simulink model "CMU_BORG_AplysiaModularNeuromechanics"  (R2024a)
settings: Solver=ode23  StartTime=0.0  StopTime=tend  FixedStep=0.001  MaxStep=0.1  RelTol=0.00001  AbsTol=0.0001
values from neighbouring files (symbols this model uses):
  B20_0 = 0    [ParameterRecalculation.m]    (also in ReferenceGeometry_and_Initialization.m)
  B31B32_0 = 0    [GetSteadyState.m]    (also in ParameterRecalculation.m = 1; ReferenceGeometry_and_Initialization.m = 1; VaryingSeaweedStrength.m = 1)
  B38_0 = 0    [ParameterRecalculation.m]    (also in ReferenceGeometry_and_Initialization.m)
  B40B30_0 = 0    [ParameterRecalculation.m]    (also in ReferenceGeometry_and_Initialization.m)
  B40B30_offTime_0 = 0    [ParameterRecalculation.m]    (also in ReferenceGeometry_and_Initialization.m)
  B43B45_0 = 0    [ParameterRecalculation.m]    (also in ReferenceGeometry_and_Initialization.m)
  B4B5_0 = 0    [ParameterRecalculation.m]    (also in ReferenceGeometry_and_Initialization.m)
  B64_0 = 1    [GetSteadyState.m]    (also in ParameterRecalculation.m = 0; ReferenceGeometry_and_Initialization.m = 0; VaryingSeaweedStrength.m = 0)
  B6B9B3_0 = 1    [GetSteadyState.m]    (also in ParameterRecalculation.m = 0; ReferenceGeometry_and_Initialization.m = 0; VaryingSeaweedStrength.m = 0)
  B7_0 = 0    [ParameterRecalculation.m]    (also in ReferenceGeometry_and_Initialization.m)
  B8_0 = 0    [ParameterRecalculation.m]    (also in ReferenceGeometry_and_Initialization.m)
  C1_0 = 0    [ParameterRecalculation.m]    (also in ReferenceGeometry_and_Initialization.m)
  C2_0 = 0    [ParameterRecalculation.m]    (also in ReferenceGeometry_and_Initialization.m)
  C6_0 = 0    [ParameterRecalculation.m]    (also in ReferenceGeometry_and_Initialization.m)
  C_theta = C_xg/(2*pi)    [ParameterRecalculation.m]    (also in ReferenceGeometry_and_Initialization.m = 0.000813600069086)
  C_xd = C_xg    [ParameterRecalculation.m]    (also in ReferenceGeometry_and_Initialization.m = 0.005112)
  C_xg = (1/inv_C(kk))*time_scaler*force_scaler    [DampingParameterConvergence.m]    (also in ReferenceGeometry_and_Initialization.m = 0.005112)
  C_xv = C_xd    [ParameterRecalculation.m]    (also in ReferenceGeometry_and_Initialization.m = 0.005112)
  C_yg = C_xg    [ParameterRecalculation.m]    (also in ReferenceGeometry_and_Initialization.m = 0.005112)
  CBI2_0 = 0    [ParameterRecalculation.m]    (also in ReferenceGeometry_and_Initialization.m)
  CBI3_0 = 0    [GetSteadyState.m]    (also in ParameterRecalculation.m = 1; ReferenceGeometry_and_Initialization.m = 1; VaryingSeaweedStrength.m = 1)
  CBI3_refractory_0 = 0    [ParameterRecalculation.m]    (also in ReferenceGeometry_and_Initialization.m)
  CBI3_stimOFF_0 = 0    [ParameterRecalculation.m]    (also in ReferenceGeometry_and_Initialization.m)
  CBI3_stimON_0 = 0    [ParameterRecalculation.m]    (also in ReferenceGeometry_and_Initialization.m)
  CBI4_0 = 0    [ParameterRecalculation.m]    (also in ReferenceGeometry_and_Initialization.m)
  E1_params = [AE10,TE10,tau_E1,L0_E1,Lmax_E1]    [ParameterRecalculation.m]    (also in ReferenceGeometry_and_Initialization.m)
  E2_params = [AE20,TE20,tau_E2,L0_E2,Lmax_E2]    [ParameterRecalculation.m]    (also in ReferenceGeometry_and_Initialization.m)
  E6_params = [AE60,TE60,tau_E6,L0_E6,Lmax_E6]    [ParameterRecalculation.m]    (also in ReferenceGeometry_and_Initialization.m)
  FE1_max = force_scaler*0.2    [ParameterRecalculation.m]    (also in ReferenceGeometry_and_Initialization.m = 0.048)
  FE2_max = FE1_max    [ParameterRecalculation.m]    (also in ReferenceGeometry_and_Initialization.m = 0.048)
  FE6_max = FE1_max    [ParameterRecalculation.m]    (also in ReferenceGeometry_and_Initialization.m = 0.048)
  FHinge_max = force_scaler*0.292    [ParameterRecalculation.m]    (also in ReferenceGeometry_and_Initialization.m = 0.07008)
  FI1d_max = force_scaler*3.2    [ParameterRecalculation.m]    (also in ReferenceGeometry_and_Initialization.m = 0.768)
  FI1v_max = FI1d_max    [ParameterRecalculation.m]    (also in ReferenceGeometry_and_Initialization.m = 0.768)
  FI2_max = force_scaler*1    [ParameterRecalculation.m]    (also in ReferenceGeometry_and_Initialization.m = 0.24)
  FI3_ant_max = force_scaler*0.1    [ParameterRecalculation.m]    (also in ReferenceGeometry_and_Initialization.m = 0.024)
  FI3_max = force_scaler*3    [ParameterRecalculation.m]    (also in ReferenceGeometry_and_Initialization.m = 0.72)
  FI4_max = force_scaler*0.9    [ParameterRecalculation.m]    (also in ReferenceGeometry_and_Initialization.m = 0.216)
  fixation_type = 0    [GetSteadyState.m]    (also in ModelController.m; VaryingSeaweedStrength.m)
  grasperR = 1    [ReferenceGeometry_and_Initialization.m]
  H_lumen = mean([L_jaw,L_LG]) / R_ref    [ReferenceGeometry_and_Initialization.m]
  Hinge_params = [A_hinge0,T_hinge0,tau_hinge,L0_hinge,Lmax_hinge]    [ParameterRecalculation.m]    (also in ReferenceGeometry_and_Initialization.m)
  I1d_params = [AI1d0,TI1d0,tau_I1d,L0_I1d,Lmax_I1d]    [ParameterRecalculation.m]    (also in ReferenceGeometry_and_Initialization.m)
  I1v_params = [AI1v0,TI1v0,tau_I1v,L0_I1v,Lmax_I1v]    [ParameterRecalculation.m]    (also in ReferenceGeometry_and_Initialization.m)
  I2_params = [AI20,TI20,tau_I2_ingestive,tau_I2_egestive,L0_I2,Lmax_I2]    [ParameterRecalculation.m]    (also in ReferenceGeometry_and_Initialization.m)
  I3_params = [AI30,TI30,tau_I3]    [ParameterRecalculation.m]    (also in ReferenceGeometry_and_Initialization.m)
  I3ant_params = [AI3_ant0,TI3_ant0,tau_I3ant]    [ParameterRecalculation.m]    (also in ReferenceGeometry_and_Initialization.m)
  I4_params = [AI40,TI40,tau_I4]    [ParameterRecalculation.m]    (also in ReferenceGeometry_and_Initialization.m)
  K_const = force_scaler*0.5    [ParameterRecalculation.m]    (also in ReferenceGeometry_and_Initialization.m = 0.12)
  K_Eso = force_scaler*0.01    [ParameterRecalculation.m]    (also in ReferenceGeometry_and_Initialization.m = 0.0024)
  K_H = force_scaler*2    [ParameterRecalculation.m]    (also in ReferenceGeometry_and_Initialization.m = 0.48)
  L0_eso = abs(xd0)    [ReferenceGeometry_and_Initialization.m]
  L0_H = 0    [ReferenceGeometry_and_Initialization.m]
  L0_I1d = L1d0    [ParameterRecalculation.m]    (also in ReferenceGeometry_and_Initialization.m)
  L0_I1v = L1v0    [ParameterRecalculation.m]    (also in ReferenceGeometry_and_Initialization.m)
  L_head = 0.82*tracing_scale_factor    [ReferenceGeometry_and_Initialization.m]
  MCC_0 = 1    [DampingParameterConvergence.m]    (also in ModelController.m; ParameterRecalculation.m = 0; ReferenceGeometry_and_Initialization.m = 0)
  params = param_vec    [ParameterRecalculation.m]    (also in ReferenceGeometry_and_Initialization.m)
  seaweed_strength = 1e6    (= 1000000)    [ModelController.m]    (also in VaryingSeaweedStrength.m = seaweed_strength_vec(ind))
  sens_chemical_lips = 0    [GetSteadyState.m]    (also in ModelController.m = 1; VaryingSeaweedStrength.m = 1)
  sens_mechanical_grasper = 1    [GetSteadyState.m]    (also in ModelController.m = 0; VaryingSeaweedStrength.m)
  sens_mechanical_lips = 1    [GetSteadyState.m]    (also in ModelController.m; VaryingSeaweedStrength.m)
  t_switch_chem_lips = 1e6    (= 1000000)    [GetSteadyState.m]    (also in ModelController.m = 54; VaryingSeaweedStrength.m)
  t_switch_fixation = 1e6    (= 1000000)    [GetSteadyState.m]    (also in ModelController.m = 30; VaryingSeaweedStrength.m = 4)
  t_switch_mech_grasp = 1e6    (= 1000000)    [GetSteadyState.m]    (also in ModelController.m = 10; VaryingSeaweedStrength.m)
  t_switch_mech_lips = 1e6    (= 1000000)    [GetSteadyState.m]    (also in ModelController.m; VaryingSeaweedStrength.m)
  theta_fg = buccal_mass_data(7)    [PlotModel.m]    (also in ReferenceGeometry_and_Initialization.m = -(head_outline{4,"Angle"} - head_outline{3,"Angle"})*(pi/180)
  theta_g0 = (180-(head_outline{3,"Angle"} + rot_global +5))*(pi/180)    [ReferenceGeometry_and_Initialization.m]
  theta_H = buccal_mass_data(6)    [PlotModel.m]    (also in ReferenceGeometry_and_Initialization.m = pi + theta_H_tilde - theta_g0)
  time_scaler = 1    [DampingParameterConvergence.m]    (also in ReferenceGeometry_and_Initialization.m = 1.065)
  ukg = 0.95*usg    (= 0.95)    [ParameterRecalculation.m]    (also in ReferenceGeometry_and_Initialization.m)
  ukh = 0.75*ush    (= 0.75)    [ParameterRecalculation.m]    (also in ReferenceGeometry_and_Initialization.m)
  usg = 1    [ParameterRecalculation.m]    (also in ReferenceGeometry_and_Initialization.m)
  ush = 1    [ParameterRecalculation.m]    (also in ReferenceGeometry_and_Initialization.m)
  xd0 = L_head - L1d0    [ReferenceGeometry_and_Initialization.m]
  xg0 = L_head + L_CG * cosd(a_CG) + 0.3    [ReferenceGeometry_and_Initialization.m]
  xh0 = 0    [ReferenceGeometry_and_Initialization.m]
  xv0 = L_head - L1v0    [ReferenceGeometry_and_Initialization.m]
  yg0 = L_CG * sind(a_CG) + 0.4    [ReferenceGeometry_and_Initialization.m]
(part 4 of 4)

== matlab function CMU_BORG_AplysiaModularNeuromechanics/Neural Model Module Webster-Wood et al. 1/MATLAB Function ==
  data: CBI3_stimOFF output; CBI3_refractory output; B40B30 output; Time input; time_scaler input; MCC output; stim_CBI2_old input; stim_B4B5_old input; sens_mechanical_lips_old input; sens_chemical_lips_old input; sens_mechanical_grasper_old input; CBI3_stimOFF_old input; CBI3_refractory_old input; B40B30_old input; CBI2 output; MCC_old input; CBI2_old input; CBI3_stimON_old input; CBI4_old input; B64_old input; B4B5_old input; B20_old input; B40B30_offTime input; CBI3_old input; B31B32_old input; P_I4_old input; x_gh input; CBI3_stimON output; CBI4 output; B64 output; B4B5 output; B20 output; B40B30_offTime output; B8 output; B38 output; B6B9B3 output; CBI3 output; B31B32 output; B7 output; params input
function [CBI3_stimOFF, CBI3_refractory, B40B30, MCC, CBI2, CBI3_stimON, CBI4, B64, B4B5, B20, B40B30_offTime, B8, B38, B6B9B3, CBI3, B31B32, B7]...
    = neuromechanics(Time,time_scaler, stim_CBI2_old, stim_B4B5_old, sens_mechanical_lips_old, sens_chemical_lips_old, sens_mechanical_grasper_old,...
    CBI3_stimOFF_old, CBI3_refractory_old, B40B30_old, MCC_old, CBI2_old, CBI3_stimON_old, ...
    CBI4_old, B64_old, B4B5_old, B20_old, B40B30_offTime, CBI3_old, B31B32_old, ...
    P_I4_old, x_gh, params)

    % All time related values were changed from step-number-dependent to
    % actual simulation time dependent for compatibility with variable
    % time-step solvers. --MB

    %% Parameter definition based on the params vector
    thresh_B31_bite_off =            params(1) ;  % retraction level at which to turn I2 back on
    thresh_B64_bite_protract =       params(2) ; % protraction level at which to turn I3 on (once I2 turns off)
    thresh_B31_bite_on =             params(3) ;  % protraction level at which to turn I2 off
    thresh_B7_bite_protract =        params(4) ;  % protraction level at which to turn the hinge on
    thresh_B7_bite_pressure =        params(5) ;   % pressure level at which B7 turns on
    thresh_B6B9B3_bite_pressure =    params(6) ;  % pressure threshold needed before I3 turns on 
    thresh_B31_pressure_bite =       params(7) ;
    
    thresh_B64_swallow_protract =    params(8) ;  % protraction level above which to turn on I3
    thresh_B31_swallow_off =         params(9) ; % retraction level at which to turn I2 back on 
    thresh_B31_swallow_on =          params(10) ;
    thresh_B6B9B3_swallow_pressure = params(11) ;
    thresh_B38_retract =             params(12) ;
    thresh_B31_pressure_swallow =    params(13) ;
    
    % rejection params
    thresh_B64_reject_protract =     params(14) ;
    thresh_B4B5_protract =           params(15) ;
    thresh_B31_reject_off =          params(16) ;
    thresh_B31_reject_on =           params(17) ;
    thresh_B7_reject_protract =      params(18) ;
    thresh_B7_reject_pressure =      params(19) ;   % pressure level at which B7 turns on
    thresh_B6B9B3_reject_pressure =  params(20) ;
    thresh_B31_pressure_reject =     params(21) ;
    refractory_CBI3 = params(22) ;
    
    postActivityExcitation_B40B30 = params(23);

    %switches
    use_hypothesized_connections = 1; %1 = yes, 0 = no

%% Update Metacerebral cell: 
                % assume here feeding arousal continues
                % indefinitely, once started. 
                %{
                MCC is active IF
                    General Food arousal is on
                %}

                MCC = MCC_old;    
    %% Update CBI-2
    
    %CBI2 - updated 6/7/2020
    %with hypothesized connections from B4/B5
    %%%%% MJB 5/27/2025 The second row of the condition (for rejection) was
    %%%%% missing the negation in front of the chemical lip stimulation.
    if (use_hypothesized_connections ==1)
         CBI2 = (stim_CBI2_old==0)*... if electrode above CBI-2 is off, do this:
             MCC_old*(~B64_old)*( (sens_mechanical_lips_old && sens_chemical_lips_old &&(~sens_mechanical_grasper_old)) || ...
                                  (sens_mechanical_grasper_old &&(~sens_chemical_lips_old)) || ...
                                  (B4B5_old>=2) )+...
             (stim_CBI2_old==1);
    else
    %without hypothesized connections from B4/B5
        CBI2 = (stim_CBI2_old==0)*... if electrode above CBI-2 is off, do this:
            MCC_old*(~B64_old)*((sens_mechanical_lips_old && sens_chemical_lips_old &&(~sens_mechanical_grasper_old))||(sens_mechanical_grasper_old&&(~sens_chemical_lips_old)))+...
            (stim_CBI2_old==1);
    end

    
    %% Update CBI-3
    
            % requires stimuli_mech_last AND stimuli_chem_last
        %{
        CBI3 is active IF
            MCC is on
            AND
            Mechanical Simulation at Lips
            AND
            Chemical Stimulation at Lips
            AND
            B4/B5 is NOT firing strongly
            AND
            CBI3 is NOT in a refractory period
        %}

        %CBI3 can experieince a refractory period following strong inhibition from B4/B5
        %check if a refractory period is occuring

    %modified to only turn on refreactory after the strong stimulation
    
        CBI3_refractory = CBI3_refractory_old;
        CBI3_stimOFF = CBI3_stimOFF_old;
        CBI3_stimON = CBI3_stimON_old;
            
        if((B4B5_old>=2) && (CBI3_stimON_old==0))
           CBI3_stimON = Time;   
           %CBI3_refractory = 1;
        end
        

        if ((CBI3_stimON_old ~=0) && (B4B5_old<2))
           CBI3_refractory = 1;
           CBI3_stimOFF = Time;  
           CBI3_stimON = 0;    
        end
        

        if(CBI3_refractory && Time<(CBI3_stimOFF + refractory_CBI3))
           CBI3_refractory = 1; 
        else
            CBI3_stimOFF = 0;
            CBI3_refractory = 0; 
        end


        %CBI3 - updated 6/7/2020    
        %with hypothesized connections from B4/B5    
        if (use_hypothesized_connections ==1)
            CBI3 = MCC_old*(sens_mechanical_lips_old*sens_chemical_lips_old)*((B4B5_old<2))*(~CBI3_refractory);   
        else
        %without hypothesized connections from B4/B5  
            CBI3 = MCC_old*(sens_mechanical_lips_old*sens_chemical_lips_old); 
        end
    %% Update CBI4 - added 2/27/2020
    %{
    CBI4 is active IF  mediates swallowing and rejection
        MCC is on
        AND
            (Mechanical Stimulation at Lips
            OR
            Chemical Stimulation at Lips)
        AND
        Mechanical Stimulation in grasper
    %}
    CBI4 = MCC_old*(sens_mechanical_lips_old || sens_chemical_lips_old)*sens_mechanical_grasper_old;
    
    %% Update B64
    % list of inputs
    % Protraction threshold excites
    % grasper pressure excites - still figuring out how to implement
    % retraction threshold inhibits
    % B31/32 inhibits

    %If there is mechanical and chemical stimuli at the lips and there is
    %seaweed in the grasper -> swallow

    %If there is mechanical and chemical stimuli at the lips and there is
    %NOT seaweed in the grasper -> bite

    %If there is not chemical stimuli at the lips but there is mechanical
    %stimuli ->reject

    %{
    B64 is active IF
        MCC is on
        AND
        IF CBI3 is active (ingestion)
            IF mechanical stimulation is in grasper (swallowing)
                Relative Grasper Position is Greater than B64 Swallowing Protraction threshold
            IF mechanical stimulation is NOT in grasper (biting)
                Relative Grasper Position is Greater than B64 Biting Protraction threshold
        IF CBI3 is NOT active (rejection)
            Relative Grasper Position is Greater than B64 Rejection Protraction threshold
        AND
        B31/B32 is NOT active
        AND
        IF CBI3 is active (ingestion)
            IF mechanical stimulation is in grasper (swallowing)
                NOT (Relative Grasper Position is less than B64 Swallow Retraction threshold)
            IF mechanical stimulation is NOT in grasper (biting)
                NOT(Relative Grasper Position is less than B64 Biting Retraction threshold)
        IF CBI3 is NOT active (rejection)
            NOT(Relative Grasper Position is less than B64 Rejection Retraction threshold)
    %}

    B64_proprioception = (CBI3_old*(... % checks protraction threshold - original 0.5
                                    (  sens_mechanical_grasper_old *(x_gh>thresh_B64_swallow_protract))||...
                                    ((~sens_mechanical_grasper_old)*(x_gh>thresh_B64_bite_protract))))...
                                ||...
                                    ((~CBI3_old)                   *(x_gh>thresh_B64_reject_protract));

    %B64
    B64 = (MCC_old*(~B31B32_old)*B64_proprioception); % update B64
%% Update B4/B5: 
    %{
    B4/B5 is active IF
        MCC is ON
        AND
        IF stimulating electrode is off
            Strongly firing IF CBI3 is NOT active (rejection)
                AND
                B64 is active (retraction)
                AND
                Relative grasper position is greater than B4/B5 threshold (early retraction)
            weakly firing IF CBI3 is active (ingestion)
                AND
                B64 is active (retraction)
                AND
                mechanical stimulation is in grasper (swallowing)
        If stimulating electrode is on
            Activity is set to 2 to designate strong firing
    %}

    %B4B5
    B4B5 = MCC_old*...
                ((~stim_B4B5_old)*... % when B4/B5 electrode is off
                    (2*(~CBI3_old)*...% if egestion
                        B64_old*(x_gh>thresh_B4B5_protract)) +... 
                    ((CBI3_old)*(sens_mechanical_grasper_old)*B64_old))... % if swallowing
        +2*stim_B4B5_old; % when B4/B5 electrode is on (and +1) then turn B4/B5 on to "emergency" mode
    
 %% Update B20 - updated 2/27/2020
    % Not active if CB1-3 is on (strongly inhibited)
    %excited by CBI2 but excitation is weaker than inhibition from CBI3
    %{
    (CBI2 is active
        OR	
        CBI4 is active
        OR
        B63 (B31/32) is active)
            AND
            CBI3 is NOT active
            AND
            B64 is NOT active
    %}
    B20 = MCC_old*((CBI2_old || CBI4_old) || B31B32_old)*(~CBI3_old)*(~B64_old);

%% Update B40/B30
    %{
    B40/B30 is active IF
        MCC is ON
        AND
        (CBI2 is active
        OR 
        CBI4 is active
        OR 
        B63 (B31/32) is active)
        AND 
        B64 is not active
    %}

    % B30/B40 have a fast inhibitory and slow excitatory connection with
    % B8a/b. To accomodate this, we track when B30/B40 goes from a active
    % state to a quiescent state 

    B40B30 = MCC_old*((CBI2_old || CBI4_old) || B31B32_old)*(~B64_old);

    %check if B30/B40 has gone from active to quiescent
    if((B40B30_old == 1) && (B40B30==0))
       B40B30_offTime = Time;
    end
%% Update B31/B32: -updated 2/27/2020
                % activated if grasper retracted enough, inhibited if
                % pressure exceeds a threshold or grasper is protracted far enough
                %{
                B31/B32 is active IF
                    MCC is ON
                    AND
                    IF CBI3 is active (ingestion)
                        B64 is NOT active (protraction)
                        AND
                            Graper pressure is less than half of its maximum (open)
                            OR
                            CBI2 is active (biting)
                        AND
                        IF B31/B32 is NOT firing (switching to protraction)
                            The relative grasper position is less than the retraction threshold
                        IF B31/B32 is firing (protraction)
                            The relative grasper position is less than the protraction threshold
                    IF CBI3 is NOT active (rejection)
                        B64 is NOT active (protraction)
                        AND
                        Grasper Pressure is greater than a quarter of the maximum (closing or closed)
                        AND
                            CBI2 is active
                            OR
                            CBI4 is active
                        AND
                        IF B31/B32 is NOT firing (switching to protraction)
                            The relative grasper position is less than the retraction threshold
                        IF B31/B32 is firing (protraction)
                            The relative grasper position is less than the protraction threshold
                %}

                %B31/B32s thresholds may vary for different behaviors. These are set
                %here
                if (sens_mechanical_grasper_old && CBI3_old) %swallowing
                    on_thresh = thresh_B31_swallow_on;
                    off_thresh = thresh_B31_swallow_off;
                    press_thresh = thresh_B31_pressure_swallow;
                elseif (sens_mechanical_grasper_old && (~CBI3_old)) %rejection
                    on_thresh = thresh_B31_reject_on;
                    off_thresh = thresh_B31_reject_off;
                    press_thresh = thresh_B31_pressure_reject;
                else %biting
                    on_thresh = thresh_B31_bite_on;
                    off_thresh = thresh_B31_bite_off;
                    press_thresh = thresh_B31_pressure_bite;
                end

                B31B32 = MCC_old*(...
                    CBI3_old*... %if ingestion
                        ((~B64_old)*((P_I4_old<(press_thresh))||CBI2_old)*... 
                            ((~B31B32_old)*(x_gh<off_thresh)+...
                               B31B32_old *(x_gh<on_thresh)))+...
                  (~CBI3_old)*... %if egestion
                        ((~B64_old)*(P_I4_old>(press_thresh))*(CBI2_old||CBI4_old)*...
                            ((~B31B32_old)*(x_gh<off_thresh)+...
                               B31B32_old *(x_gh<on_thresh))));

%% Update B6/B9/B3: 
    % activate once pressure is high enough in ingestion, or low enough in
    % rejection
    %{
    NEW VERSION:
    B6/B9/B3 is active IF
        MCC is active
        AND
        B4/B5 is NOT firing strongly
        AND
        IF CBI3 is active (ingestion)
            B64 is active (retraction)
            AND
            Grasper pressure is greater than B6/B3/B9 pressure threshold (closed)
        IF CBI3 is not active (rejection)
            B64 is active (retraction)
            AND
            Grasper pressure is less than B6/B3/B9 pressure threshold (open)
    %}

    %B6/B9/B3
    B6B9B3 = MCC_old*B64_old*(~(B4B5_old>=2))*(...
                    (CBI3_old && ~sens_mechanical_grasper_old)*... biting
                        (P_I4_old>thresh_B6B9B3_bite_pressure)...
                    +...
                    (CBI3_old && sens_mechanical_grasper_old)*... swallowing
                        (P_I4_old>thresh_B6B9B3_swallow_pressure)...
                    +...
                    (~CBI3_old)*... rejection
                        (~(P_I4_old>thresh_B6B9B3_reject_pressure)));

%% Update B8a/b
    % active if excitation from B6/B9/B3 plus protracted
    % sensory feedback exceeds threshold of 1.9, and not inhibited by
    % either B31/B32 or by sensory feedback from being retracted. If B4/B5 is
    % highly excited (activation level is 2 instead of just 1) then shut
    % down B8a/b.
    %{
    B8a/b is active IF
        MCC is on
        AND
            B64 is active
            OR
            B40/B30 is NOT active
            OR
            B20 is active
        AND
        B4/B5 is not active
        AND
            B20 is active
            OR
            B31/B32 is NOT active
    %}

    %B8a/b recieves slow exitatory input from B30/B40 functionally this
    %causes strong firing immediatly following B30/B40 cessation in biting
    %and swallowing
    if(B40B30_old==0 && Time<(B40B30_offTime+postActivityExcitation_B40B30)) %%%%%%%%Changed 'TimeStep' to 0.01 - ASL
        B40B30_excite = 1; 
    else
        B40B30_excite = 0; 
    end

    %B8a/b - updated 5/25/2020   
    B8 = MCC_old*(~(B4B5_old>=2))*(...%B4/5 inhibits when strongly active
                CBI3_old*(... % if ingestion
                    B20_old || (B40B30_excite)*(~B31B32_old))+...
                (~CBI3_old)*(... % if rejection
                    B20_old));                     

%% Update B7 - ONLY ACTIVE DURING EGESTION and BITING
    % turn on as you get to peak protraction
    %in biting this has a threshold that it stops applying effective force -
    %biomechanics
    %{
    B7 is active IF
        ((CBI3 is NOT active (rejection)
        OR
        There is mechanical stimulation in mouth
        AND
            (The relative position of the grasper is greater than the rejection protraction threshold
            OR
            Grasper pressure is very high) (closed))
        OR
        (CBI3 is active
        AND
        There is NOT mechanical stimulation in mouth (biting)
        AND
            (The relative position of the grasper is greater than the bite protraction threshold
            OR
            Grasper pressure is very high) (closed))
    %}
    B7 = MCC_old*( ...
                      (((~CBI3_old) ||  (sens_mechanical_grasper_old))*((x_gh>=thresh_B7_reject_protract)||(P_I4_old>(thresh_B7_reject_pressure)))) + ...
                      (  (CBI3_old  && (~sens_mechanical_grasper_old))*((x_gh>=thresh_B7_bite_protract)  ||(P_I4_old>(thresh_B7_bite_pressure)))) ...
                      );                    

%% Update B38: 
    % If already active, remain active until protracted past
    % 0.5.  If inactive, become active if retracted to 0.1 or further. 
    %{
    B38 is active IF
        MCC is ON
        AND
        mechanical stimulation in the grasper (swallowing or rejection)
        AND
        IF CBI3 is active (ingestion)
            Relative grasper position is less than B38 ingestion threshold
        IF CBI3 is not active (rejection)
            Turn off B38
    %}

    %B38

    B38 = MCC_old*(sens_mechanical_grasper_old)*(...
        (CBI3_old)*(... % if CBI3 active do the following:
            ((x_gh)<thresh_B38_retract)));
